simulink library "dlbsBlockProduct"  (R2025b)
settings: Solver=VariableStepAuto  StartTime=0.0  StopTime=10.0  RelTol=1e-3
libraries: dlbsBlockInsertGradientGF x2, dlbsBlockExtractGradientGF x1
settings Model: Creator=lt6037  LastModifiedBy=lt6037

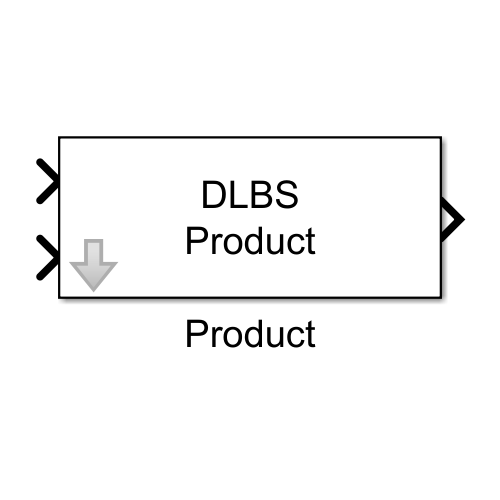
[thumbnail: Simulink's stored preview of the top-level diagram]
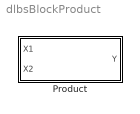
== system dlbsBlockProduct ==
  Product : Subsystem
      mask help: Computes element-wise multiplication of two input tensors.
      mask Help: web("dlbsHelpBlockProduct.html")
      mask Display: fprintf("DLBS\nProduct")

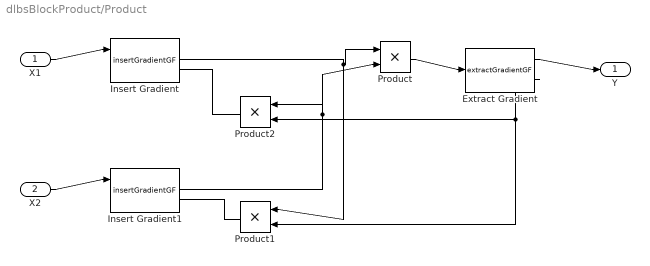
== system dlbsBlockProduct/Product ==
  X1 : Inport
  X2 : Inport  Port=2
  Extract Gradient : dlbsBlockExtractGradientGF/extractGradientGF
  Insert Gradient : dlbsBlockInsertGradientGF/insertGradientGF
  Insert Gradient1 : dlbsBlockInsertGradientGF/insertGradientGF
  Product : Product
  Product1 : Product
  Product2 : Product
  Y : Outport
  wires:
  Insert Gradient/1 -> Product1/1, Product/1
  Insert Gradient1/1 -> Product2/1, Product/2
  Product1/1 -> Insert Gradient1/2
  Extract Gradient/2 -> Product1/2, Product2/2
  Product2/1 -> Insert Gradient/2
  Product/1 -> Extract Gradient/1
  X1/1 -> Insert Gradient/1
  X2/1 -> Insert Gradient1/1
  Extract Gradient/1 -> Y/1
